simulink model "MCU_Fault"  (R2022b)
settings: Solver=FixedStepDiscrete  StartTime=0.0  StopTime=10.0  FixedStep=1e-4  RelTol=1e-3
values from neighbouring files (symbols this model uses):
  C_Fault_CntDectiontime_u32 = 0.0    [MCU_FaultDiag_Datadictionary.sldd]    (also in MCU_Fault_Datadictionary_objects.m = myPackage.Parameter; MCU_Fault_Datadictionary_objects.sldd)
  C_Fault_IaConfirmCnt_u16 = 0.0    [MCU_FaultDiag_Datadictionary.sldd]    (also in MCU_Fault_Datadictionary_objects.m = myPackage.Parameter; MCU_Fault_Datadictionary_objects.sldd)
  C_Fault_IbConfirmCnt_u16 = 0.0    [MCU_FaultDiag_Datadictionary.sldd]    (also in MCU_Fault_Datadictionary_objects.m = myPackage.Parameter; MCU_Fault_Datadictionary_objects.sldd)
  C_Fault_IbLimit_s32 = 0.0    [MCU_FaultDiag_Datadictionary.sldd]    (also in MCU_Fault_Datadictionary_objects.m = myPackage.Parameter; MCU_Fault_Datadictionary_objects.sldd)
  C_Fault_IcConfirmCnt_u16 = 0.0    [MCU_FaultDiag_Datadictionary.sldd]    (also in MCU_Fault_Datadictionary_objects.m = myPackage.Parameter; MCU_Fault_Datadictionary_objects.sldd)
  C_Fault_IcLimit_s32 = 0.0    [MCU_FaultDiag_Datadictionary.sldd]    (also in MCU_Fault_Datadictionary_objects.m = myPackage.Parameter; MCU_Fault_Datadictionary_objects.sldd)
  C_Fault_IphaseLimitStart_s32 = 0.0    [MCU_FaultDiag_Datadictionary.sldd]    (also in MCU_Fault_Datadictionary_objects.m = myPackage.Parameter; MCU_Fault_Datadictionary_objects.sldd)
  C_Fault_MotorTempSensor_i16 = 0.0    [MCU_FaultDiag_Datadictionary.sldd]    (also in MCU_Fault_Datadictionary_objects.m = myPackage.Parameter; MCU_Fault_Datadictionary_objects.sldd)
  C_Fault_SpdUpFaultConfirmCnt_u16 = 0.0    [MCU_FaultDiag_Datadictionary.sldd]    (also in MCU_Fault_Datadictionary_objects.m = myPackage.Parameter; MCU_Fault_Datadictionary_objects.sldd)
  C_Fault_SpdUpLimitStart_i16 = 0.0    [MCU_FaultDiag_Datadictionary.sldd]    (also in MCU_Fault_Datadictionary_objects.m = myPackage.Parameter; MCU_Fault_Datadictionary_objects.sldd)
  C_Fault_SpdUpLimitStop_i16 = 0.0    [MCU_FaultDiag_Datadictionary.sldd]    (also in MCU_Fault_Datadictionary_objects.m = myPackage.Parameter; MCU_Fault_Datadictionary_objects.sldd)
  C_Fault_SpdUpWarnConfirmCnt_u16 = 0.0    [MCU_FaultDiag_Datadictionary.sldd]    (also in MCU_Fault_Datadictionary_objects.m = myPackage.Parameter; MCU_Fault_Datadictionary_objects.sldd)
  C_Fault_TigbtCircutConfirmCnt_u16 = 0.0    [MCU_FaultDiag_Datadictionary.sldd]    (also in MCU_Fault_Datadictionary_objects.m = myPackage.Parameter; MCU_Fault_Datadictionary_objects.sldd)
  C_Fault_TigbtCircutConfirmTh_u16 = 0.0    [MCU_FaultDiag_Datadictionary.sldd]    (also in MCU_Fault_Datadictionary_objects.m = myPackage.Parameter; MCU_Fault_Datadictionary_objects.sldd)
  C_Fault_TigbtCircutFaultEn_u8 = 0.0    [MCU_FaultDiag_Datadictionary.sldd]    (also in MCU_Fault_Datadictionary_objects.m = myPackage.Parameter; MCU_Fault_Datadictionary_objects.sldd)
  C_Fault_TigbtLimitStart_i16 = 0.0    [MCU_FaultDiag_Datadictionary.sldd]    (also in MCU_Fault_Datadictionary_objects.m = myPackage.Parameter; MCU_Fault_Datadictionary_objects.sldd)
  C_Fault_TigbtLimitStop_i16 = 0.0    [MCU_FaultDiag_Datadictionary.sldd]    (also in MCU_Fault_Datadictionary_objects.m = myPackage.Parameter; MCU_Fault_Datadictionary_objects.sldd)
  C_Fault_TigbtOverConfirmCnt_u16 = 0.0    [MCU_FaultDiag_Datadictionary.sldd]    (also in MCU_Fault_Datadictionary_objects.m = myPackage.Parameter; MCU_Fault_Datadictionary_objects.sldd)
  C_Fault_TigbtWarnConfirmCnt_u16 = 0.0    [MCU_FaultDiag_Datadictionary.sldd]    (also in MCU_Fault_Datadictionary_objects.m = myPackage.Parameter; MCU_Fault_Datadictionary_objects.sldd)
  C_Fault_TmotorCircutConfirmCnt_u16 = 0.0    [MCU_FaultDiag_Datadictionary.sldd]    (also in MCU_Fault_Datadictionary_objects.m = myPackage.Parameter; MCU_Fault_Datadictionary_objects.sldd)
  C_Fault_TmotorCircutConfirmTh_u16 = 0.0    [MCU_FaultDiag_Datadictionary.sldd]    (also in MCU_Fault_Datadictionary_objects.m = myPackage.Parameter; MCU_Fault_Datadictionary_objects.sldd)
  C_Fault_TmotorCircutFaultEn_u8 = 0.0    [MCU_FaultDiag_Datadictionary.sldd]    (also in MCU_Fault_Datadictionary_objects.m = myPackage.Parameter; MCU_Fault_Datadictionary_objects.sldd)
  C_Fault_TmotorLimitStart_i16 = 0.0    [MCU_FaultDiag_Datadictionary.sldd]    (also in MCU_Fault_Datadictionary_objects.m = myPackage.Parameter; MCU_Fault_Datadictionary_objects.sldd)
  C_Fault_TmotorLimitStop_i16 = 0.0    [MCU_FaultDiag_Datadictionary.sldd]    (also in MCU_Fault_Datadictionary_objects.m = myPackage.Parameter; MCU_Fault_Datadictionary_objects.sldd)
  C_Fault_TmotorOverConfirmCnt_u16 = 0.0    [MCU_FaultDiag_Datadictionary.sldd]    (also in MCU_Fault_Datadictionary_objects.m = myPackage.Parameter; MCU_Fault_Datadictionary_objects.sldd)
  C_Fault_TmotorWarnConfirmCnt_u16 = 0.0    [MCU_FaultDiag_Datadictionary.sldd]    (also in MCU_Fault_Datadictionary_objects.m = myPackage.Parameter; MCU_Fault_Datadictionary_objects.sldd)
  C_Fault_UdcLoFaultConfirmCnt_u16 = 0.0    [MCU_FaultDiag_Datadictionary.sldd]    (also in MCU_Fault_Datadictionary_objects.m = myPackage.Parameter; MCU_Fault_Datadictionary_objects.sldd)
  C_Fault_UdcLoWarnConfirmCnt_u16 = 0.0    [MCU_FaultDiag_Datadictionary.sldd]    (also in MCU_Fault_Datadictionary_objects.m = myPackage.Parameter; MCU_Fault_Datadictionary_objects.sldd)
  C_Fault_UdcUpFaultConfirmCnt_u16 = 0.0    [MCU_FaultDiag_Datadictionary.sldd]    (also in MCU_Fault_Datadictionary_objects.m = myPackage.Parameter; MCU_Fault_Datadictionary_objects.sldd)
  C_Fault_UdcUpWarnConfirmCnt_u16 = 0.0    [MCU_FaultDiag_Datadictionary.sldd]    (also in MCU_Fault_Datadictionary_objects.m = myPackage.Parameter; MCU_Fault_Datadictionary_objects.sldd)
undefined symbols (not defined in the file or in its folder): AB_SAMPLE, ABC_SAMPLE, AC_SAMPLE, BC_SAMPLE, ParamCfg_LaValueDefault_u16, ParamCfg_SampleMode_u16, VEHICLE
libraries: simulink x30
(part 1 of 2)
settings Model: DataDictionary=MCU_Fault_Datadictionary_objects.sldd  Creator=ZYH  LastModifiedBy=ZYH
settings OptimizationCC: DefaultParameterBehavior=Inlined  EnhancedBackFolding=on  PassReuseOutputArgsAs=Individual arguments  ZeroExternalMemoryAtStartup=off  ZeroInternalMemoryAtStartup=off  OptimizeBlockOrder=speed  DifferentSizesBufferReuse=on  OptimizationCustomize=off  EfficientTunableParamExpr=on
settings DebuggingCC: ParameterTunabilityLossMsg=error
settings SFSimCC: MATLABDynamicMemAlloc=off
settings RTWCC: Description=Embedded Coder  SystemTargetFile=ert.tlc  GenCodeOnly=on  TemplateMakefile=ert_default_tmf
settings CodeAppCC: ForceParamTrailComments=on  IgnoreCustomStorageClasses=off  OperatorAnnotations=on  SimulinkDataObjDesc=on  SFDataObjDesc=on  InsertBlockDesc=on
settings ERTTargetCC: TargetLangStandard=C99 (ISO)  GenerateSampleERTMain=on  InlinedParameterPlacement=NonHierarchical  ERTCustomFileTemplate=example_file_process.tlc

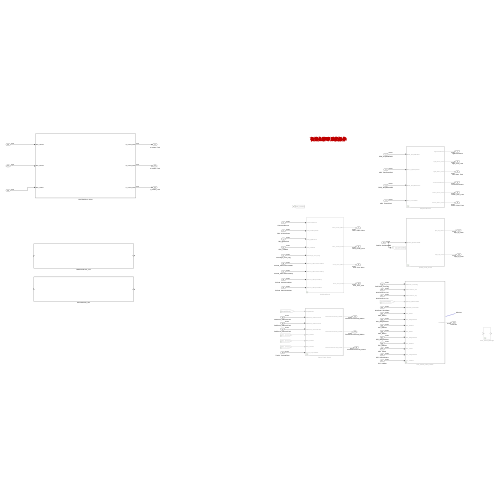
[thumbnail: Simulink's stored preview of the top-level diagram]
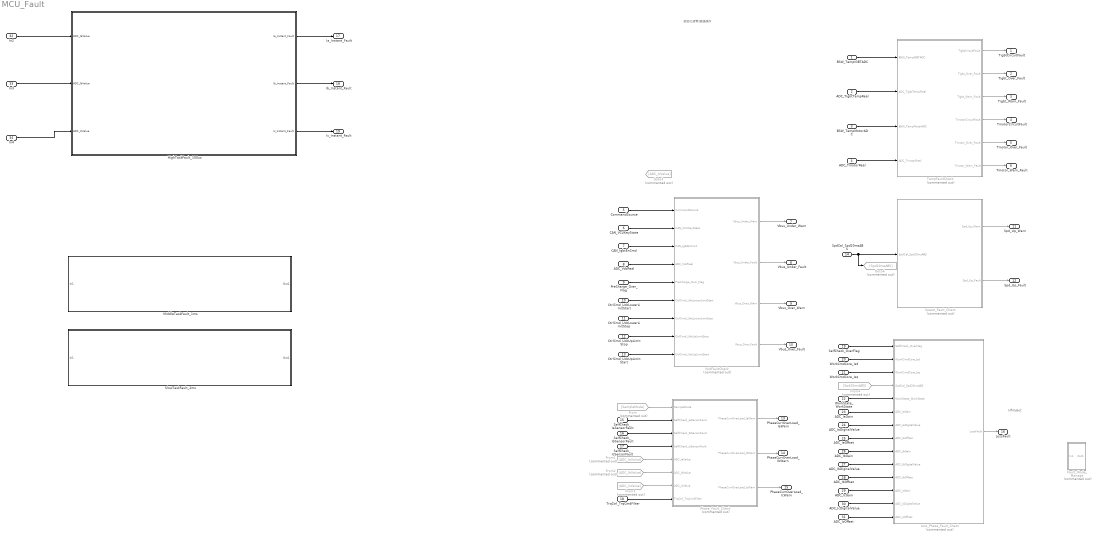
== system MCU_Fault ==
  note: 初始化清零/赋值操作
  note: HfiInJect
  BSW_TempIGBTADC : Inport
  ADC_TigbtTempReal : Inport  Port=2
  BSW_TempMotorADC : Inport  Port=3
  ADC_TmotorReal : Inport  Port=4
  CommandSource : Inport  Port=5
  CAN_VCUKeyState : Inport  Port=6
  CAN_IgbtEnCmd : Inport  Port=7
  ADC_VdcReal : Inport  Port=8
  PreCharge_Over_Flag : Inport  Port=9
  CtrlCmd_UdcLowerLimitStart : Inport  Port=10
  CtrlCmd_UdcLowerLimitStop : Inport  Port=11
  CtrlCmd_UdcUpLimitStop : Inport  Port=12
  CtrlCmd_UdcUpLimitStart : Inport  Port=13
  SpdCal_Spd20msABS : Inport  Port=14
  SelfCheck_IaSensorFault : Inport  Port=15
  SelfCheck_IbSensorFault : Inport  Port=16
  SelfCheck_IcSensorFault : Inport  Port=17
  TrqCtrl_TrqCmdFilter : Inport  Port=18
  SelfCheck_OverFlag : Inport  Port=19
  WorkCmdCore_Isd : Inport  Port=20
  WorkCmdCore_Isq : Inport  Port=21
  WorkState_WorkState : Inport  Port=22
  ADC_IaGain : Inport  Port=23
  ADC_IaDigitalValue : Inport  Port=24
  ADC_IaOffset : Inport  Port=25
  ADC_IbGain : Inport  Port=26
  ADC_IbDigitalValue : Inport  Port=27
  ADC_IbOffset : Inport  Port=28
  ADC_IcGain : Inport  Port=29
  ADC_IcDigitalValue : Inport  Port=30
  ADC_IcOffset : Inport  Port=31
  In2 : Inport  Port=32
  In3 : Inport  Port=33
  In4 : Inport  Port=34
  Fault_Mode_Manage : Subsystem  Commented=on
  From : From  Commented=on  GotoTag=SampleMode
  From1 : From  Commented=on  GotoTag=ADC_IaValue
  From2 : From  Commented=on  GotoTag=ADC_IbValue
  From3 : From  Commented=on  GotoTag=ADC_IcValue
  From4 : From  Commented=on  GotoTag=Spd20msABS
  Goto3 : Goto  Commented=on  GotoTag=ADC_IcValue
  Goto4 : Goto  Commented=on  GotoTag=Spd20msABS
  HighTaskFault_100us : Subsystem
  Lost_Phase_Fault_Check : Subsystem  Commented=on  TreatAsAtomicUnit=on
  MiddleTaskFault_1ms : Subsystem
  Phase_Fault_Check : Subsystem  Commented=on  TreatAsAtomicUnit=on
  SlowTaskFault_2ms : Subsystem
  Speed_Fault_Check : Subsystem  Commented=on  TreatAsAtomicUnit=on
  TempFaultCheck : Subsystem  Commented=on  TreatAsAtomicUnit=on
      settings: RTWSystemCode=Nonreusable function
  VoltFaultCheck : Subsystem  Commented=on
      settings: RTWSystemCode=Nonreusable function
  TigbtCircuitFault : Outport
  Tigbt_Over_Fault : Outport  Port=2
  Tigbt_Warn_Fault : Outport  Port=3
  TmotorCircuitFault : Outport  Port=4
  Tmotor_Over_Fault : Outport  Port=5
  Tmotor_Warn_Fault : Outport  Port=6
  Vbus_Under_Warn : Outport  Port=7
  Vbus_Under_Fault : Outport  Port=8
  Vbus_Over_Warn : Outport  Port=9
  Vbus_Over_Fault : Outport  Port=10
  Spd_Up_Warn : Outport  Port=11
  Spd_Up_Fault : Outport  Port=12
  PhaseCurrOverLoad_IaWarn : Outport  Port=13
  PhaseCurrOverLoad_IbWarn : Outport  Port=14
  PhaseCurrOverLoad_IcWarn : Outport  Port=15
  LossFault : Outport  Port=16
  Ia_Instant_Fault : Outport  Port=17
  Ib_Instant_Fault : Outport  Port=18
  Ic_Instant_Fault : Outport  Port=19
  wires:
  BSW_TempIGBTADC/1 -> TempFaultCheck/1(BSW_TempIGBTADC)
  ADC_TmotorReal/1 -> TempFaultCheck/4(ADC_TmotorReal)
  ADC_TigbtTempReal/1 -> TempFaultCheck/2(ADC_TigbtTempReal)
  BSW_TempMotorADC/1 -> TempFaultCheck/3(BSW_TempMotorADC)
  TempFaultCheck/1(TigbtCircuitFault) -> TigbtCircuitFault/1
  TempFaultCheck/2(Tigbt_Over_Fault) -> Tigbt_Over_Fault/1
  TempFaultCheck/3(Tigbt_Warn_Fault) -> Tigbt_Warn_Fault/1
  TempFaultCheck/4(TmotorCircuitFault) -> TmotorCircuitFault/1
  TempFaultCheck/5(Tmotor_Over_Fault) -> Tmotor_Over_Fault/1
  TempFaultCheck/6(Tmotor_Warn_Fault) -> Tmotor_Warn_Fault/1
  CommandSource/1 -> VoltFaultCheck/1(CommandSource)
  CAN_VCUKeyState/1 -> VoltFaultCheck/2(CAN_VCUKeyState)
  CAN_IgbtEnCmd/1 -> VoltFaultCheck/3(CAN_IgbtEnCmd)
  ADC_VdcReal/1 -> VoltFaultCheck/4(ADC_VdcReal)
  PreCharge_Over_Flag/1 -> VoltFaultCheck/5(PreCharge_Over_Flag)
  CtrlCmd_UdcLowerLimitStart/1 -> VoltFaultCheck/6(CtrlCmd_UdcLowerLimitStart)
  CtrlCmd_UdcLowerLimitStop/1 -> VoltFaultCheck/7(CtrlCmd_UdcLowerLimitStop)
  CtrlCmd_UdcUpLimitStop/1 -> VoltFaultCheck/8(CtrlCmd_UdcUpLimitStop)
  CtrlCmd_UdcUpLimitStart/1 -> VoltFaultCheck/9(CtrlCmd_UdcUpLimitStart)
  VoltFaultCheck/1(Vbus_Under_Warn) -> Vbus_Under_Warn/1
  VoltFaultCheck/2(Vbus_Under_Fault) -> Vbus_Under_Fault/1
  VoltFaultCheck/3(Vbus_Over_Warn) -> Vbus_Over_Warn/1
  VoltFaultCheck/4(Vbus_Over_Fault) -> Vbus_Over_Fault/1
  SpdCal_Spd20msABS/1 -> Speed_Fault_Check/1(SpdCal_Spd20msABS), Goto4/1
  Speed_Fault_Check/1(Spd_Up_Warn) -> Spd_Up_Warn/1
  Speed_Fault_Check/2(Spd_Up_Fault) -> Spd_Up_Fault/1
  SelfCheck_IaSensorFault/1 -> Phase_Fault_Check/2(SelfCheck_IaSensorFault)
  SelfCheck_IbSensorFault/1 -> Phase_Fault_Check/3(SelfCheck_IbSensorFault)
  SelfCheck_IcSensorFault/1 -> Phase_Fault_Check/4(SelfCheck_IcSensorFault)
  From/1 -> Phase_Fault_Check/1(SampleMode)
  From1/1 -> Phase_Fault_Check/5(ADC_IaValue)
  From2/1 -> Phase_Fault_Check/6(ADC_IbValue)
  From3/1 -> Phase_Fault_Check/7(ADC_IcValue)
  TrqCtrl_TrqCmdFilter/1 -> Phase_Fault_Check/8(TrqCtrl_TrqCmdFilter)
  Phase_Fault_Check/1(PhaseCurrOverLoad_IaWarn) -> PhaseCurrOverLoad_IaWarn/1
  Phase_Fault_Check/2(PhaseCurrOverLoad_IbWarn) -> PhaseCurrOverLoad_IbWarn/1
  Phase_Fault_Check/3(PhaseCurrOverLoad_IcWarn) -> PhaseCurrOverLoad_IcWarn/1
  SelfCheck_OverFlag/1 -> Lost_Phase_Fault_Check/1(SelfCheck_OverFlag)
  WorkCmdCore_Isd/1 -> Lost_Phase_Fault_Check/2(WorkCmdCore_Isd)
  WorkCmdCore_Isq/1 -> Lost_Phase_Fault_Check/3(WorkCmdCore_Isq)
  From4/1 -> Lost_Phase_Fault_Check/4(SpdCal_Spd20msABS)
  WorkState_WorkState/1 -> Lost_Phase_Fault_Check/5(WorkState_WorkState)
  ADC_IaGain/1 -> Lost_Phase_Fault_Check/6(ADC_IaGain)
  ADC_IaDigitalValue/1 -> Lost_Phase_Fault_Check/7(ADC_IaDigitalValue)
  ADC_IaOffset/1 -> Lost_Phase_Fault_Check/8(ADC_IaOffset)
  ADC_IbGain/1 -> Lost_Phase_Fault_Check/9(ADC_IbGain)
  ADC_IbDigitalValue/1 -> Lost_Phase_Fault_Check/10(ADC_IbDigitalValue)
  ADC_IbOffset/1 -> Lost_Phase_Fault_Check/11(ADC_IbOffset)
  ADC_IcGain/1 -> Lost_Phase_Fault_Check/12(ADC_IcGain)
  ADC_IcDigitalValue/1 -> Lost_Phase_Fault_Check/13(ADC_IcDigitalValue)
  ADC_IcOffset/1 -> Lost_Phase_Fault_Check/14(ADC_IcOffset)
  Lost_Phase_Fault_Check/1(LossFault) -> LossFault/1
  In3/1 -> HighTaskFault_100us/2(ADC_IbValue)
  In4/1 -> HighTaskFault_100us/3(ADC_IcValue)
  In2/1 -> HighTaskFault_100us/1(ADC_IaValue)
  HighTaskFault_100us/3(Ic_Instant_Fault) -> Ic_Instant_Fault/1
  HighTaskFault_100us/2(Ib_Instant_Fault) -> Ib_Instant_Fault/1
  HighTaskFault_100us/1(Ia_Instant_Fault) -> Ia_Instant_Fault/1

== system MCU_Fault/Fault_Mode_Manage ==
  In1 : Inport
  Out1 : Outport
  wires:
  In1/1 -> Out1/1

== system MCU_Fault/HighTaskFault_100us ==
  ADC_IaValue : Inport
  ADC_IbValue : Inport  Port=2
  ADC_IcValue : Inport  Port=3
  Constant : Constant  Value=ParamCfg_SampleMode_u16
  InterruptFaultCheck_100us : Subsystem  TreatAsAtomicUnit=on
      settings: RTWSystemCode=Nonreusable function
  Ia_Instant_Fault : Outport
  Ib_Instant_Fault : Outport  Port=2
  Ic_Instant_Fault : Outport  Port=3
  wires:
  ADC_IcValue/1 -> InterruptFaultCheck_100us/4(ADC_IcValue)
  ADC_IbValue/1 -> InterruptFaultCheck_100us/3(ADC_IbValue)
  ADC_IaValue/1 -> InterruptFaultCheck_100us/2(ADC_IaValue)
  InterruptFaultCheck_100us/1(Ia_Instant_Fault) -> Ia_Instant_Fault/1
  InterruptFaultCheck_100us/2(Ib_Instant_Fault) -> Ib_Instant_Fault/1
  InterruptFaultCheck_100us/3(Ic_Instant_Fault) -> Ic_Instant_Fault/1
  Constant/1 -> InterruptFaultCheck_100us/1(SampleMode)

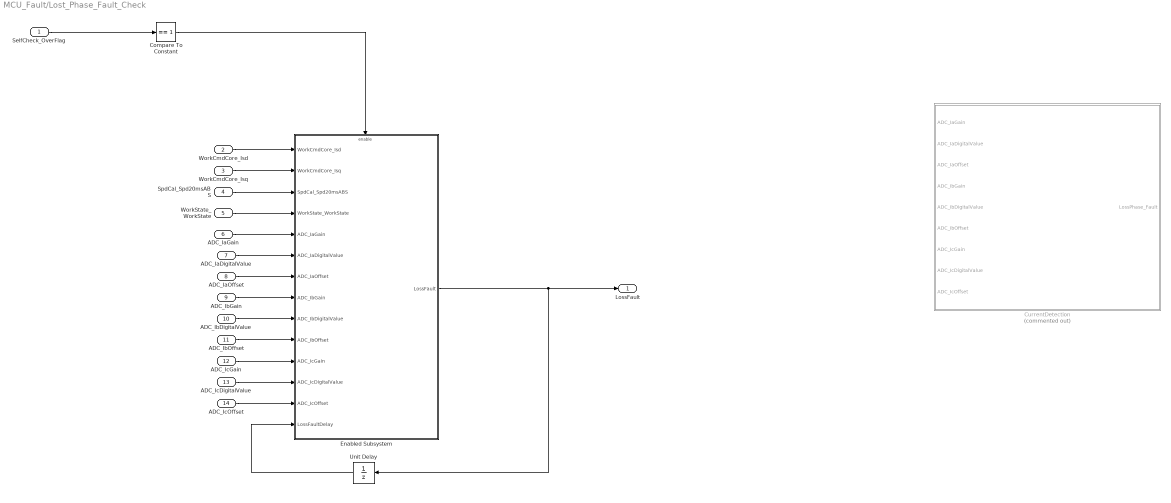
== system MCU_Fault/Lost_Phase_Fault_Check ==
  SelfCheck_OverFlag : Inport
  WorkCmdCore_Isd : Inport  Port=2
  WorkCmdCore_Isq : Inport  Port=3
  SpdCal_Spd20msABS : Inport  Port=4
  WorkState_WorkState : Inport  Port=5
  ADC_IaGain : Inport  Port=6
  ADC_IaDigitalValue : Inport  Port=7
  ADC_IaOffset : Inport  Port=8
  ADC_IbGain : Inport  Port=9
  ADC_IbDigitalValue : Inport  Port=10
  ADC_IbOffset : Inport  Port=11
  ADC_IcGain : Inport  Port=12
  ADC_IcDigitalValue : Inport  Port=13
  ADC_IcOffset : Inport  Port=14
  Compare To Constant : simulink/Logic and Bit Operations/Compare To Constant  relop===  const=1  OutDataTypeStr=boolean
  CurrentDetection : Subsystem  Commented=on
  Enabled Subsystem : Subsystem  TreatAsAtomicUnit=on
  Unit Delay : UnitDelay  SampleTime=-1  HasFrameUpgradeWarning=on
  LossFault : Outport
  wires:
  SelfCheck_OverFlag/1 -> Compare To Constant/1
  Compare To Constant/1 -> Enabled Subsystem/Enable
  Enabled Subsystem/1(LossFault) -> LossFault/1, Unit Delay/1
  Unit Delay/1 -> Enabled Subsystem/14(LossFaultDelay)
  WorkCmdCore_Isd/1 -> Enabled Subsystem/1(WorkCmdCore_Isd)
  WorkCmdCore_Isq/1 -> Enabled Subsystem/2(WorkCmdCore_Isq)
  SpdCal_Spd20msABS/1 -> Enabled Subsystem/3(SpdCal_Spd20msABS)
  WorkState_WorkState/1 -> Enabled Subsystem/4(WorkState_WorkState)
  ADC_IaGain/1 -> Enabled Subsystem/5(ADC_IaGain)
  ADC_IaDigitalValue/1 -> Enabled Subsystem/6(ADC_IaDigitalValue)
  ADC_IaOffset/1 -> Enabled Subsystem/7(ADC_IaOffset)
  ADC_IbGain/1 -> Enabled Subsystem/8(ADC_IbGain)
  ADC_IbDigitalValue/1 -> Enabled Subsystem/9(ADC_IbDigitalValue)
  ADC_IbOffset/1 -> Enabled Subsystem/10(ADC_IbOffset)
  ADC_IcGain/1 -> Enabled Subsystem/11(ADC_IcGain)
  ADC_IcDigitalValue/1 -> Enabled Subsystem/12(ADC_IcDigitalValue)
  ADC_IcOffset/1 -> Enabled Subsystem/13(ADC_IcOffset)

== system MCU_Fault/MiddleTaskFault_1ms ==
  In1 : Inport
  Out1 : Outport
  wires:
  In1/1 -> Out1/1

== system MCU_Fault/Phase_Fault_Check ==
  SampleMode : Inport
  SelfCheck_IaSensorFault : Inport  Port=2
  SelfCheck_IbSensorFault : Inport  Port=3
  SelfCheck_IcSensorFault : Inport  Port=4
  ADC_IaValue : Inport  Port=5
  ADC_IbValue : Inport  Port=6
  ADC_IcValue : Inport  Port=7
  TrqCtrl_TrqCmdFilter : Inport  Port=8
  Compare To Zero : simulink/Logic and Bit Operations/Compare To Zero  relop===  OutDataTypeStr=boolean
  Compare To Zero1 : simulink/Logic and Bit Operations/Compare To Zero  relop===  OutDataTypeStr=boolean
  Compare To Zero2 : simulink/Logic and Bit Operations/Compare To Zero  relop===  OutDataTypeStr=boolean
  Logical Operator3 : Logic  Inputs=3  AllPortsSameDT=off  OutDataTypeStr=boolean
  Subsystem : Subsystem
  PhaseCurrOverLoad_IaWarn : Outport
  PhaseCurrOverLoad_IbWarn : Outport  Port=2
  PhaseCurrOverLoad_IcWarn : Outport  Port=3
  wires:
  SelfCheck_IaSensorFault/1 -> Compare To Zero/1  "M_Fault_IaSensorFault_u8"
  SelfCheck_IbSensorFault/1 -> Compare To Zero1/1  "M_Fault_IbSensorFault_u8"
  SelfCheck_IcSensorFault/1 -> Compare To Zero2/1  "M_Fault_IcSensorFault_u8"
  Compare To Zero/1 -> Logical Operator3/1
  Compare To Zero1/1 -> Logical Operator3/2
  Compare To Zero2/1 -> Logical Operator3/3
  SampleMode/1 -> Subsystem/1(SampleMode)
  Logical Operator3/1 -> Subsystem/Enable
  ADC_IaValue/1 -> Subsystem/2(ADC_IaValue)
  ADC_IbValue/1 -> Subsystem/3(ADC_IbValue)
  ADC_IcValue/1 -> Subsystem/4(ADC_IcValue)
  TrqCtrl_TrqCmdFilter/1 -> Subsystem/5(TrqCtrl_TrqCmdFilter)  "M_Fault_TrqCmdFilter_s32"
  Subsystem/1(PhaseCurrOverLoad_IaWarn) -> PhaseCurrOverLoad_IaWarn/1
  Subsystem/2(PhaseCurrOverLoad_IbWarn) -> PhaseCurrOverLoad_IbWarn/1
  Subsystem/3(PhaseCurrOverLoad_IcWarn) -> PhaseCurrOverLoad_IcWarn/1

== system MCU_Fault/SlowTaskFault_2ms ==
  In1 : Inport
  Out1 : Outport
  wires:
  In1/1 -> Out1/1

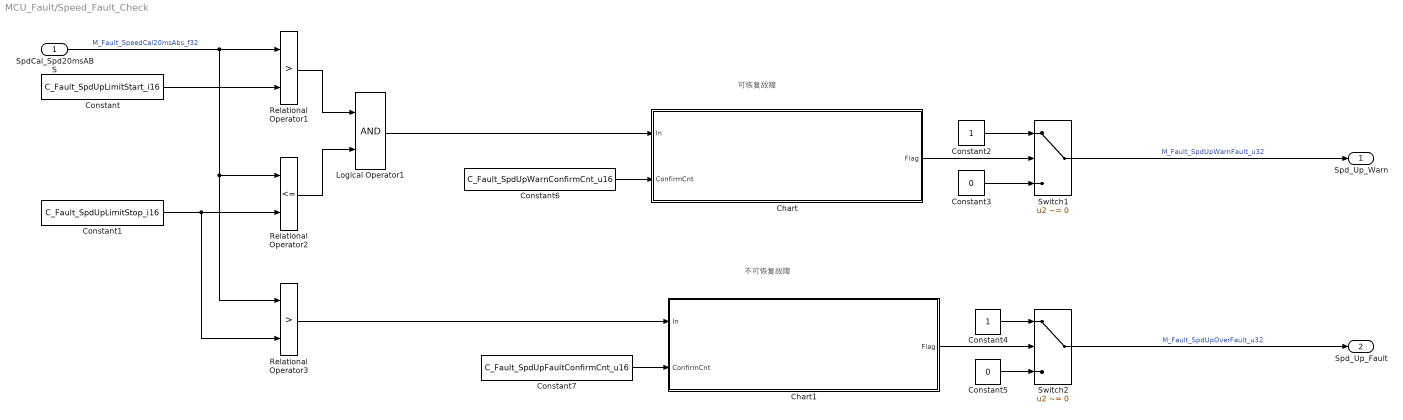
== system MCU_Fault/Speed_Fault_Check ==
  note: 不可恢复故障
  note: 可恢复故障
  SpdCal_Spd20msABS : Inport
  Chart : Stateflow chart  TreatAsAtomicUnit=on
  Chart1 : Stateflow chart  TreatAsAtomicUnit=on
  Constant : Constant  Value=C_Fault_SpdUpLimitStart_i16
  Constant1 : Constant  Value=C_Fault_SpdUpLimitStop_i16
  Constant2 : Constant  OutDataTypeStr=uint32
  Constant3 : Constant  Value=0  OutDataTypeStr=uint32
  Constant4 : Constant  OutDataTypeStr=uint32
  Constant5 : Constant  Value=0  OutDataTypeStr=uint32
  Constant6 : Constant  Value=C_Fault_SpdUpWarnConfirmCnt_u16
  Constant7 : Constant  Value=C_Fault_SpdUpFaultConfirmCnt_u16
  Logical Operator1 : Logic  AllPortsSameDT=off  OutDataTypeStr=boolean
  Relational Operator1 : RelationalOperator  Operator=>  OutDataTypeStr=boolean  RndMeth=Simplest  InputSameDT=off
  Relational Operator2 : RelationalOperator  Operator=<=  OutDataTypeStr=boolean  RndMeth=Simplest  InputSameDT=off
  Relational Operator3 : RelationalOperator  Operator=>  OutDataTypeStr=boolean  RndMeth=Simplest  InputSameDT=off
  Switch1 : Switch  Criteria=u2 ~= 0  SaturateOnIntegerOverflow=off  InputSameDT=off
  Switch2 : Switch  Criteria=u2 ~= 0  SaturateOnIntegerOverflow=off  InputSameDT=off
  Spd_Up_Warn : Outport
  Spd_Up_Fault : Outport  Port=2
  wires:
  Logical Operator1/1 -> Chart/1(In)
  Switch2/1 -> Spd_Up_Fault/1  "M_Fault_SpdUpOverFault_u32"
  Relational Operator3/1 -> Chart1/1(In)
  Constant5/1 -> Switch2/3
  Switch1/1 -> Spd_Up_Warn/1  "M_Fault_SpdUpWarnFault_u32"
  Chart1/1(Flag) -> Switch2/2
  Constant4/1 -> Switch2/1
  Relational Operator1/1 -> Logical Operator1/1
  Constant7/1 -> Chart1/2(ConfirmCnt)
  Constant1/1 -> Relational Operator3/2, Relational Operator2/2
  Constant6/1 -> Chart/2(ConfirmCnt)
  Constant3/1 -> Switch1/3
  SpdCal_Spd20msABS/1 -> Relational Operator3/1, Relational Operator2/1, Relational Operator1/1  "M_Fault_SpeedCal20msAbs_f32"
  Chart/1(Flag) -> Switch1/2
  Constant2/1 -> Switch1/1
  Constant/1 -> Relational Operator1/2
  Relational Operator2/1 -> Logical Operator1/2

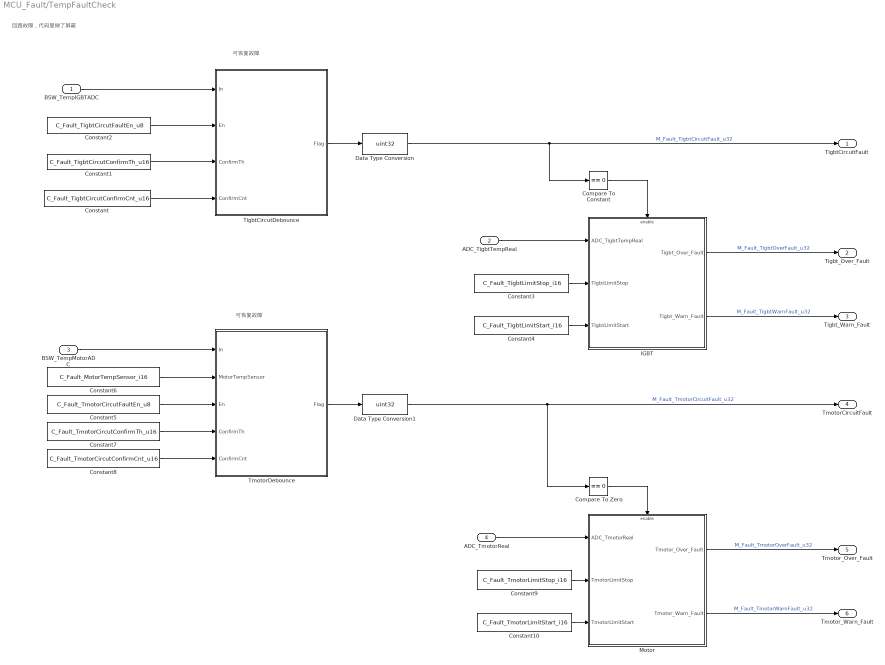
== system MCU_Fault/TempFaultCheck ==
  note: 回路故障，代码里做了屏蔽
  note: 可恢复故障
  note: 可恢复故障
  BSW_TempIGBTADC : Inport
  ADC_TigbtTempReal : Inport  Port=2
  BSW_TempMotorADC : Inport  Port=3
  ADC_TmotorReal : Inport  Port=4
  Compare To Constant : simulink/Logic and Bit Operations/Compare To Constant  relop===  const=0  OutDataTypeStr=boolean
  Compare To Zero : simulink/Logic and Bit Operations/Compare To Zero  relop===  OutDataTypeStr=boolean
  Constant : Constant  Value=C_Fault_TigbtCircutConfirmCnt_u16  OutDataTypeStr=uint16
  Constant1 : Constant  Value=C_Fault_TigbtCircutConfirmTh_u16  OutDataTypeStr=uint16
  Constant10 : Constant  Value=C_Fault_TmotorLimitStart_i16  OutDataTypeStr=int16
  Constant2 : Constant  Value=C_Fault_TigbtCircutFaultEn_u8  OutDataTypeStr=uint8
  Constant3 : Constant  Value=C_Fault_TigbtLimitStop_i16  OutDataTypeStr=int16
  Constant4 : Constant  Value=C_Fault_TigbtLimitStart_i16  OutDataTypeStr=int16
  Constant5 : Constant  Value=C_Fault_TmotorCircutFaultEn_u8  OutDataTypeStr=uint8
  Constant6 : Constant  Value=C_Fault_MotorTempSensor_i16  OutDataTypeStr=int16
  Constant7 : Constant  Value=C_Fault_TmotorCircutConfirmTh_u16  OutDataTypeStr=uint16
  Constant8 : Constant  Value=C_Fault_TmotorCircutConfirmCnt_u16  OutDataTypeStr=uint16
  Constant9 : Constant  Value=C_Fault_TmotorLimitStop_i16  OutDataTypeStr=int16
  Data Type Conversion : DataTypeConversion  OutDataTypeStr=uint32  SaturateOnIntegerOverflow=off  RndMeth=Floor
  Data Type Conversion1 : DataTypeConversion  OutDataTypeStr=uint32  SaturateOnIntegerOverflow=off  RndMeth=Floor
  IGBT : Subsystem  TreatAsAtomicUnit=on
  Motor : Subsystem  TreatAsAtomicUnit=on
  TigbtCircutDebounce : Stateflow chart  TreatAsAtomicUnit=on
      settings: PortSchema="{\"entries\":[{\"content\":{\"sides\":[{\"content\":{\"connectorIds\":[\"In2\",\"In4\",\"In3\",\"In1\"]},\"type\":\"ConnectorPlacement.EquallySpacedRectSide\",\"uuid\":\"cb643c20-0648-4de0-95a0-2dc0cea02081\"},{\"content\":{\"connectorIds\":[\"Out1\"],\"side\":\"RIGHT\"},\"type\":\"ConnectorPlacement.EquallySpacedRectSide\",\"uuid\":\"2b2785c0-bbb5-46d9-9c97-4314d513a69a\"},{\"content\":{\"connectorIds\":[],\"side\":\"TOP\"},\"type\":\"ConnectorPlacement.EquallySpacedRectSide\",\"uuid\":\"79ac1ab1-637b-4565-8653-1b1baa55e4cd\"}]},\"type\":\"ConnectorPlacement.EquallySpacedConnector\",\"uuid\":\"b76854ae-8754-44d0-b8b9-3a13cdedbdf9\"}],\"packageUris\":[\"http://schema.mathworks.com/mf0/Connector/R2020b\"],\"version\":\"1.0\"}"
  TmotorDebounce : Stateflow chart  TreatAsAtomicUnit=on
      settings: PortSchema="{\"entries\":[{\"content\":{\"sides\":[{\"content\":{\"connectorIds\":[\"In3\",\"In2\",\"In5\",\"In4\",\"In1\"]},\"type\":\"ConnectorPlacement.EquallySpacedRectSide\",\"uuid\":\"cb643c20-0648-4de0-95a0-2dc0cea02081\"},{\"content\":{\"connectorIds\":[\"Out1\"],\"side\":\"RIGHT\"},\"type\":\"ConnectorPlacement.EquallySpacedRectSide\",\"uuid\":\"2b2785c0-bbb5-46d9-9c97-4314d513a69a\"},{\"content\":{\"connectorIds\":[],\"side\":\"TOP\"},\"type\":\"ConnectorPlacement.EquallySpacedRectSide\",\"uuid\":\"79ac1ab1-637b-4565-8653-1b1baa55e4cd\"}]},\"type\":\"ConnectorPlacement.EquallySpacedConnector\",\"uuid\":\"b76854ae-8754-44d0-b8b9-3a13cdedbdf9\"}],\"packageUris\":[\"http://schema.mathworks.com/mf0/Connector/R2020b\"],\"version\":\"1.0\"}"
  TigbtCircuitFault : Outport
  Tigbt_Over_Fault : Outport  Port=2
  Tigbt_Warn_Fault : Outport  Port=3
  TmotorCircuitFault : Outport  Port=4
  Tmotor_Over_Fault : Outport  Port=5
  Tmotor_Warn_Fault : Outport  Port=6
  wires:
  Constant1/1 -> TigbtCircutDebounce/3(ConfirmTh)
  Constant/1 -> TigbtCircutDebounce/1(ConfirmCnt)
  Constant2/1 -> TigbtCircutDebounce/4(En)
  BSW_TempIGBTADC/1 -> TigbtCircutDebounce/2(In)
  TigbtCircutDebounce/1(Flag) -> Data Type Conversion/1
  Data Type Conversion/1 -> Compare To Constant/1, TigbtCircuitFault/1  "M_Fault_TigbtCircuitFault_u32"
  Compare To Constant/1 -> IGBT/Enable
  Constant3/1 -> IGBT/2(TigbtLimitStop)
  Constant4/1 -> IGBT/3(TigbtLimitStart)
  ADC_TigbtTempReal/1 -> IGBT/1(ADC_TigbtTempReal)
  IGBT/1(Tigbt_Over_Fault) -> Tigbt_Over_Fault/1  "M_Fault_TigbtOverFault_u32"
  IGBT/2(Tigbt_Warn_Fault) -> Tigbt_Warn_Fault/1  "M_Fault_TigbtWarnFault_u32"
  BSW_TempMotorADC/1 -> TmotorDebounce/3(In)
  Constant6/1 -> TmotorDebounce/2(MotorTempSensor)
  Constant5/1 -> TmotorDebounce/5(En)
  Constant8/1 -> TmotorDebounce/1(ConfirmCnt)
  Constant7/1 -> TmotorDebounce/4(ConfirmTh)
  TmotorDebounce/1(Flag) -> Data Type Conversion1/1
  Data Type Conversion1/1 -> Compare To Zero/1, TmotorCircuitFault/1  "M_Fault_TmotorCircuitFault_u32"
  Compare To Zero/1 -> Motor/Enable
  ADC_TmotorReal/1 -> Motor/1(ADC_TmotorReal)
  Constant9/1 -> Motor/2(TmotorLimitStop)
  Constant10/1 -> Motor/3(TmotorLimitStart)
  Motor/1(Tmotor_Over_Fault) -> Tmotor_Over_Fault/1  "M_Fault_TmotorOverFault_u32"
  Motor/2(Tmotor_Warn_Fault) -> Tmotor_Warn_Fault/1  "M_Fault_TmotorWarnFault_u32"

== system MCU_Fault/VoltFaultCheck ==
  note: 不做成标定量是因为
      | 代码里区分了Analog模式和其他模式下的欠过压阈值
  CommandSource : Inport
  CAN_VCUKeyState : Inport  Port=2
  CAN_IgbtEnCmd : Inport  Port=3
  ADC_VdcReal : Inport  Port=4
  PreCharge_Over_Flag : Inport  Port=5
  CtrlCmd_UdcLowerLimitStart : Inport  Port=6
  CtrlCmd_UdcLowerLimitStop : Inport  Port=7
  CtrlCmd_UdcUpLimitStop : Inport  Port=8
  CtrlCmd_UdcUpLimitStart : Inport  Port=9
  VdcLowerFaultCheck : Subsystem  TreatAsAtomicUnit=on
  VdcOverFaultCheck : Subsystem  TreatAsAtomicUnit=on
  Vbus_Under_Warn : Outport
  Vbus_Under_Fault : Outport  Port=2
  Vbus_Over_Warn : Outport  Port=3
  Vbus_Over_Fault : Outport  Port=4
  wires:
  CommandSource/1 -> VdcLowerFaultCheck/1(CommandSource)  "M_Fault_CommandSource_i16"
  CAN_VCUKeyState/1 -> VdcLowerFaultCheck/2(CAN_VCUKeyState)  "M_Fault_VCUKeyState_u16"
  CAN_IgbtEnCmd/1 -> VdcLowerFaultCheck/3(CAN_IgbtEnCmd)  "M_Fault_IgbtEnCmd_u16"
  PreCharge_Over_Flag/1 -> VdcLowerFaultCheck/4(PreCharge_Over_Flag)  "M_Fault_PrechargeOverFlg_u16"
  ADC_VdcReal/1 -> VdcOverFaultCheck/1(ADC_VdcReal), VdcLowerFaultCheck/5(ADC_VdcReal)  "M_Fault_UdcReal_s32"
  CtrlCmd_UdcLowerLimitStart/1 -> VdcLowerFaultCheck/6(CtrlCmd_UdcLowerLimitStart)  "M_Fault_UdcLowerLimitStart_s32"
  CtrlCmd_UdcLowerLimitStop/1 -> VdcLowerFaultCheck/7(CtrlCmd_UdcLowerLimitStop)  "M_Fault_UdcLowerLimitStop_s32"
  VdcLowerFaultCheck/1(Vbus_Under_Warn) -> Vbus_Under_Warn/1  "M_Fault_VdcUnderWarn_u32"
  VdcLowerFaultCheck/2(Vbus_Under_Fault) -> Vbus_Under_Fault/1  "M_Fault_VdcUnderFault_u32"
  CtrlCmd_UdcUpLimitStop/1 -> VdcOverFaultCheck/3(CtrlCmd_UdcUpLimitStop)  "M_Fault_UdcUpLimitStop_s32"
  CtrlCmd_UdcUpLimitStart/1 -> VdcOverFaultCheck/2(CtrlCmd_UdcUpLimitStart)  "M_Fault_UdcUpLimitStart_s32"
  VdcOverFaultCheck/1(Vbus_Over_Warn) -> Vbus_Over_Warn/1  "M_Fault_UdcUpWarn_u32"
  VdcOverFaultCheck/2(Vbus_Over_Fault) -> Vbus_Over_Fault/1  "M_Fault_UdcUpFault_u32"

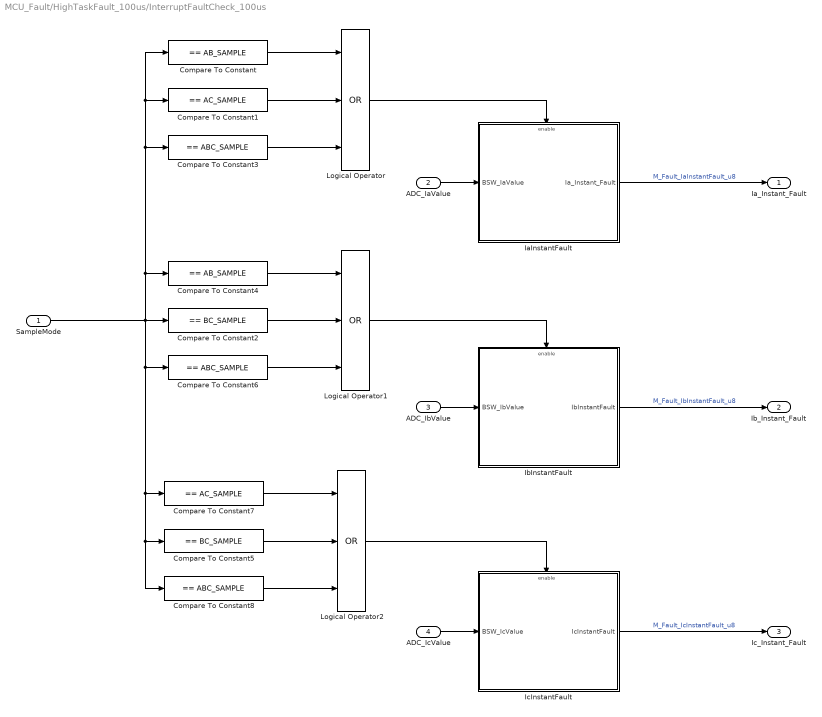
== system MCU_Fault/HighTaskFault_100us/InterruptFaultCheck_100us ==
  SampleMode : Inport
  ADC_IaValue : Inport  Port=2
  ADC_IbValue : Inport  Port=3
  ADC_IcValue : Inport  Port=4
  Compare To Constant : simulink/Logic and Bit Operations/Compare To Constant  relop===  const=AB_SAMPLE  OutDataTypeStr=boolean
  Compare To Constant1 : simulink/Logic and Bit Operations/Compare To Constant  relop===  const=AC_SAMPLE  OutDataTypeStr=boolean
  Compare To Constant2 : simulink/Logic and Bit Operations/Compare To Constant  relop===  const=BC_SAMPLE  OutDataTypeStr=boolean
  Compare To Constant3 : simulink/Logic and Bit Operations/Compare To Constant  relop===  const=ABC_SAMPLE  OutDataTypeStr=boolean
  Compare To Constant4 : simulink/Logic and Bit Operations/Compare To Constant  relop===  const=AB_SAMPLE  OutDataTypeStr=boolean
  Compare To Constant5 : simulink/Logic and Bit Operations/Compare To Constant  relop===  const=BC_SAMPLE  OutDataTypeStr=boolean
  Compare To Constant6 : simulink/Logic and Bit Operations/Compare To Constant  relop===  const=ABC_SAMPLE  OutDataTypeStr=boolean
  Compare To Constant7 : simulink/Logic and Bit Operations/Compare To Constant  relop===  const=AC_SAMPLE  OutDataTypeStr=boolean
  Compare To Constant8 : simulink/Logic and Bit Operations/Compare To Constant  relop===  const=ABC_SAMPLE  OutDataTypeStr=boolean
  IaInstantFault : Subsystem  TreatAsAtomicUnit=on
  IbInstantFault : Subsystem  TreatAsAtomicUnit=on
  IcInstantFault : Subsystem  TreatAsAtomicUnit=on
  Logical Operator : Logic  Operator=OR  Inputs=3  AllPortsSameDT=off  OutDataTypeStr=boolean
  Logical Operator1 : Logic  Operator=OR  Inputs=3  AllPortsSameDT=off  OutDataTypeStr=boolean
  Logical Operator2 : Logic  Operator=OR  Inputs=3  AllPortsSameDT=off  OutDataTypeStr=boolean
  Ia_Instant_Fault : Outport
  Ib_Instant_Fault : Outport  Port=2
  Ic_Instant_Fault : Outport  Port=3
  wires:
  SampleMode/1 -> Compare To Constant/1, Compare To Constant1/1, Compare To Constant3/1, Compare To Constant4/1, Compare To Constant8/1, Compare To Constant5/1, Compare To Constant7/1, Compare To Constant6/1, Compare To Constant2/1
  Compare To Constant/1 -> Logical Operator/1
  Compare To Constant1/1 -> Logical Operator/2
  Compare To Constant3/1 -> Logical Operator/3
  Logical Operator/1 -> IaInstantFault/Enable
  ADC_IaValue/1 -> IaInstantFault/1(BSW_IaValue)
  Compare To Constant6/1 -> Logical Operator1/3
  Compare To Constant2/1 -> Logical Operator1/2
  Compare To Constant4/1 -> Logical Operator1/1
  Logical Operator1/1 -> IbInstantFault/Enable
  ADC_IbValue/1 -> IbInstantFault/1(BSW_IbValue)
  Compare To Constant5/1 -> Logical Operator2/2
  Compare To Constant7/1 -> Logical Operator2/1
  Compare To Constant8/1 -> Logical Operator2/3
  Logical Operator2/1 -> IcInstantFault/Enable
  ADC_IcValue/1 -> IcInstantFault/1(BSW_IcValue)
  IaInstantFault/1(Ia_Instant_Fault) -> Ia_Instant_Fault/1  "M_Fault_IaInstantFault_u8"
  IbInstantFault/1(IbInstantFault) -> Ib_Instant_Fault/1  "M_Fault_IbInstantFault_u8"
  IcInstantFault/1(IcInstantFault) -> Ic_Instant_Fault/1  "M_Fault_IcInstantFault_u8"

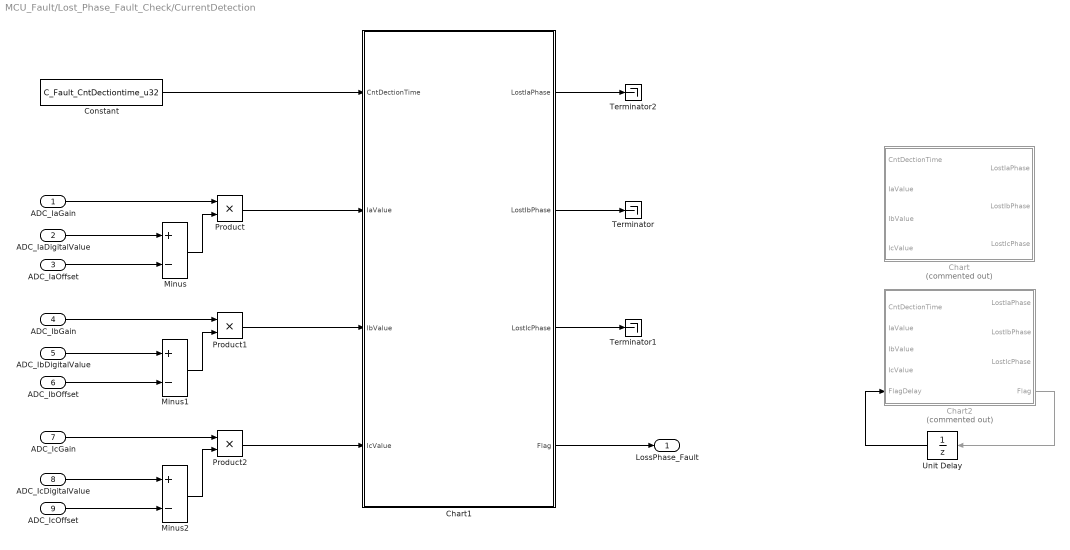
== system MCU_Fault/Lost_Phase_Fault_Check/CurrentDetection ==
  ADC_IaGain : Inport
  ADC_IaDigitalValue : Inport  Port=2
  ADC_IaOffset : Inport  Port=3
  ADC_IbGain : Inport  Port=4
  ADC_IbDigitalValue : Inport  Port=5
  ADC_IbOffset : Inport  Port=6
  ADC_IcGain : Inport  Port=7
  ADC_IcDigitalValue : Inport  Port=8
  ADC_IcOffset : Inport  Port=9
  Chart : Stateflow chart  Commented=on  TreatAsAtomicUnit=on
  Chart1 : Stateflow chart  TreatAsAtomicUnit=on
  Chart2 : Stateflow chart  Commented=on  TreatAsAtomicUnit=on
      settings: PortSchema="{\"entries\":[{\"content\":{\"sides\":[{\"content\":{\"connectorIds\":[\"In2\",\"In3\",\"In4\",\"In5\",\"In1\"]},\"type\":\"ConnectorPlacement.EquallySpacedRectSide\",\"uuid\":\"7ee51362-cc53-4c4b-bb72-7e7d7fdfa368\"},{\"content\":{\"connectorIds\":[\"Out1\",\"Out2\",\"Out3\",\"Out4\"],\"side\":\"RIGHT\"},\"type\":\"ConnectorPlacement.EquallySpacedRectSide\",\"uuid\":\"f10f55d3-9130-490d-9732-47c24a5d1591\"},{\"content\":{\"connectorIds\":[],\"side\":\"TOP\"},\"type\":\"ConnectorPlacement.EquallySpacedRectSide\",\"uuid\":\"d4ead924-d192-479a-942e-9c33d44277d2\"},{\"content\":{\"connectorIds\":[],\"side\":\"BOTTOM\"},\"type\":\"ConnectorPlacement.EquallySpacedRectSide\",\"uuid\":\"0567de3f-c1c5-4c0c-81d8-e5bcc3ace347\"}]},\"type\":\"ConnectorPlacement.EquallySpacedConnector\",\"uuid\":\"51e6a2cf-dee8-429b-a62c-1b7f30850334\"}],\"packageUris\":[\"http://schema.mathworks.com/mf0/Connector/R2020b\"],\"version\":\"1.0\"}"
  Constant : Constant  Value=C_Fault_CntDectiontime_u32
  Minus : Sum  Inputs=+-
  Minus1 : Sum  Inputs=+-
  Minus2 : Sum  Inputs=+-
  Product : Product
  Product1 : Product
  Product2 : Product
  Terminator : Terminator
  Terminator1 : Terminator
  Terminator2 : Terminator
  Unit Delay : UnitDelay  SampleTime=-1  HasFrameUpgradeWarning=on
  LossPhase_Fault : Outport
  wires:
  ADC_IaDigitalValue/1 -> Minus/1
  ADC_IaOffset/1 -> Minus/2
  ADC_IaGain/1 -> Product/1
  Minus/1 -> Product/2
  Product/1 -> Chart1/2(IaValue)
  ADC_IbDigitalValue/1 -> Minus1/1
  ADC_IbOffset/1 -> Minus1/2
  ADC_IbGain/1 -> Product1/1
  Minus1/1 -> Product1/2
  ADC_IcDigitalValue/1 -> Minus2/1
  ADC_IcOffset/1 -> Minus2/2
  ADC_IcGain/1 -> Product2/1
  Minus2/1 -> Product2/2
  Product1/1 -> Chart1/3(IbValue)
  Product2/1 -> Chart1/4(IcValue)
  Constant/1 -> Chart1/1(CntDectionTime)
  Chart1/2(LostIbPhase) -> Terminator/1
  Chart1/3(LostIcPhase) -> Terminator1/1
  Chart1/1(LostIaPhase) -> Terminator2/1
  Chart1/4(Flag) -> LossPhase_Fault/1
  Chart2/4(Flag) -> Unit Delay/1
  Unit Delay/1 -> Chart2/1(FlagDelay)

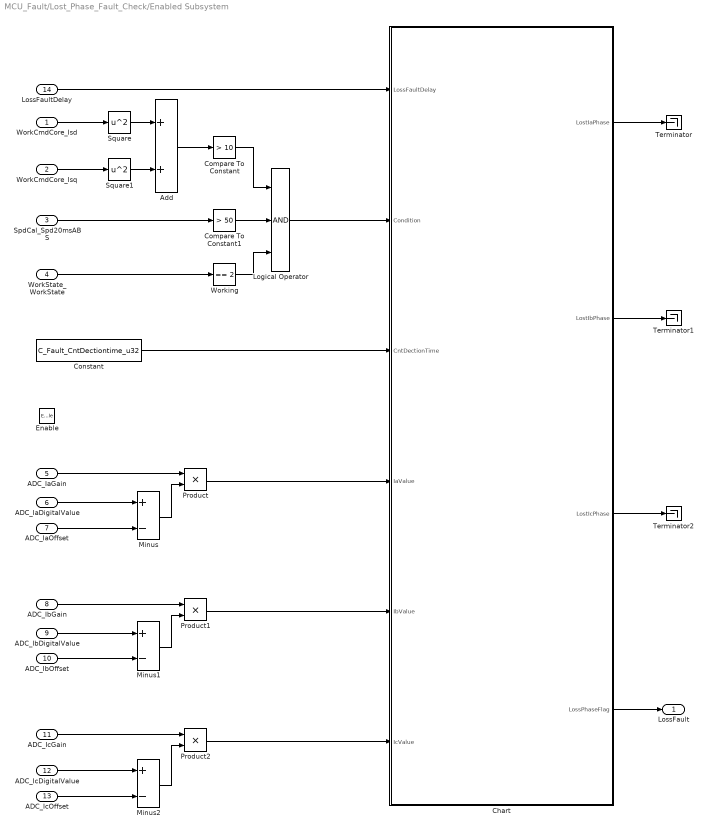
== system MCU_Fault/Lost_Phase_Fault_Check/Enabled Subsystem ==
  WorkCmdCore_Isd : Inport
  WorkCmdCore_Isq : Inport  Port=2
  SpdCal_Spd20msABS : Inport  Port=3
  WorkState_WorkState : Inport  Port=4
  ADC_IaGain : Inport  Port=5
  ADC_IaDigitalValue : Inport  Port=6
  ADC_IaOffset : Inport  Port=7
  ADC_IbGain : Inport  Port=8
  ADC_IbDigitalValue : Inport  Port=9
  ADC_IbOffset : Inport  Port=10
  ADC_IcGain : Inport  Port=11
  ADC_IcDigitalValue : Inport  Port=12
  ADC_IcOffset : Inport  Port=13
  LossFaultDelay : Inport  Port=14
  Enable : EnablePort
  Add : Sum
  Chart : Stateflow chart  TreatAsAtomicUnit=on
  Compare To Constant : simulink/Logic and Bit Operations/Compare To Constant  relop=>  const=10  OutDataTypeStr=boolean
  Compare To Constant1 : simulink/Logic and Bit Operations/Compare To Constant  relop=>  const=50  OutDataTypeStr=boolean
  Constant : Constant  Value=C_Fault_CntDectiontime_u32
  Logical Operator : Logic  Inputs=3  AllPortsSameDT=off  OutDataTypeStr=boolean
  Minus : Sum  Inputs=+-
  Minus1 : Sum  Inputs=+-
  Minus2 : Sum  Inputs=+-
  Product : Product
  Product1 : Product
  Product2 : Product
  Square : Math  Operator=square
  Square1 : Math  Operator=square
  Terminator : Terminator
  Terminator1 : Terminator
  Terminator2 : Terminator
  Working : simulink/Logic and Bit Operations/Compare To Constant  relop===  const=2  OutDataTypeStr=boolean
  LossFault : Outport
  wires:
  LossFaultDelay/1 -> Chart/1(LossFaultDelay)
  WorkCmdCore_Isd/1 -> Square/1
  WorkCmdCore_Isq/1 -> Square1/1
  Square/1 -> Add/1
  Square1/1 -> Add/2
  Add/1 -> Compare To Constant/1
  SpdCal_Spd20msABS/1 -> Compare To Constant1/1
  WorkState_WorkState/1 -> Working/1
  Compare To Constant1/1 -> Logical Operator/2
  Compare To Constant/1 -> Logical Operator/1
  Working/1 -> Logical Operator/3
  Logical Operator/1 -> Chart/2(Condition)
  Product/1 -> Chart/4(IaValue)
  Product2/1 -> Chart/6(IcValue)
  ADC_IaDigitalValue/1 -> Minus/1
  ADC_IcGain/1 -> Product2/1
  Product1/1 -> Chart/5(IbValue)
  ADC_IaOffset/1 -> Minus/2
  Minus1/1 -> Product1/2
  ADC_IaGain/1 -> Product/1
  ADC_IbOffset/1 -> Minus1/2
  ADC_IcOffset/1 -> Minus2/2
  Minus/1 -> Product/2
  ADC_IbDigitalValue/1 -> Minus1/1
  Minus2/1 -> Product2/2
  ADC_IcDigitalValue/1 -> Minus2/1
  ADC_IbGain/1 -> Product1/1
  Constant/1 -> Chart/3(CntDectionTime)
  Chart/1(LostIaPhase) -> Terminator/1
  Chart/2(LostIbPhase) -> Terminator1/1
  Chart/3(LostIcPhase) -> Terminator2/1
  Chart/4(LossPhaseFlag) -> LossFault/1

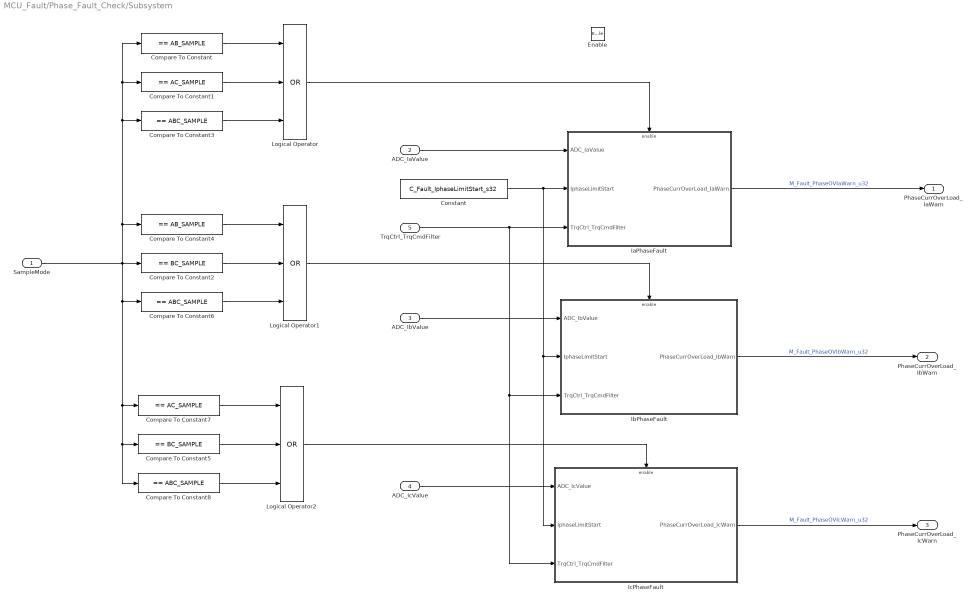
== system MCU_Fault/Phase_Fault_Check/Subsystem ==
  SampleMode : Inport
  ADC_IaValue : Inport  Port=2
  ADC_IbValue : Inport  Port=3
  ADC_IcValue : Inport  Port=4
  TrqCtrl_TrqCmdFilter : Inport  Port=5
  Enable : EnablePort
  Compare To Constant : simulink/Logic and Bit Operations/Compare To Constant  relop===  const=AB_SAMPLE  OutDataTypeStr=boolean
  Compare To Constant1 : simulink/Logic and Bit Operations/Compare To Constant  relop===  const=AC_SAMPLE  OutDataTypeStr=boolean
  Compare To Constant2 : simulink/Logic and Bit Operations/Compare To Constant  relop===  const=BC_SAMPLE  OutDataTypeStr=boolean
  Compare To Constant3 : simulink/Logic and Bit Operations/Compare To Constant  relop===  const=ABC_SAMPLE  OutDataTypeStr=boolean
  Compare To Constant4 : simulink/Logic and Bit Operations/Compare To Constant  relop===  const=AB_SAMPLE  OutDataTypeStr=boolean
  Compare To Constant5 : simulink/Logic and Bit Operations/Compare To Constant  relop===  const=BC_SAMPLE  OutDataTypeStr=boolean
  Compare To Constant6 : simulink/Logic and Bit Operations/Compare To Constant  relop===  const=ABC_SAMPLE  OutDataTypeStr=boolean
  Compare To Constant7 : simulink/Logic and Bit Operations/Compare To Constant  relop===  const=AC_SAMPLE  OutDataTypeStr=boolean
  Compare To Constant8 : simulink/Logic and Bit Operations/Compare To Constant  relop===  const=ABC_SAMPLE  OutDataTypeStr=boolean
  Constant : Constant  Value=C_Fault_IphaseLimitStart_s32
  IaPhaseFault : Subsystem  TreatAsAtomicUnit=on
  IbPhaseFault : Subsystem  TreatAsAtomicUnit=on
  IcPhaseFault : Subsystem  TreatAsAtomicUnit=on
  Logical Operator : Logic  Operator=OR  Inputs=3  AllPortsSameDT=off  OutDataTypeStr=boolean
  Logical Operator1 : Logic  Operator=OR  Inputs=3  AllPortsSameDT=off  OutDataTypeStr=boolean
  Logical Operator2 : Logic  Operator=OR  Inputs=3  AllPortsSameDT=off  OutDataTypeStr=boolean
  PhaseCurrOverLoad_IaWarn : Outport
  PhaseCurrOverLoad_IbWarn : Outport  Port=2
  PhaseCurrOverLoad_IcWarn : Outport  Port=3
  wires:
  Compare To Constant7/1 -> Logical Operator2/1
  Compare To Constant8/1 -> Logical Operator2/3
  Compare To Constant1/1 -> Logical Operator/2
  Compare To Constant/1 -> Logical Operator/1
  SampleMode/1 -> Compare To Constant/1, Compare To Constant1/1, Compare To Constant3/1, Compare To Constant4/1, Compare To Constant8/1, Compare To Constant5/1, Compare To Constant7/1, Compare To Constant6/1, Compare To Constant2/1
  Compare To Constant4/1 -> Logical Operator1/1
  Compare To Constant6/1 -> Logical Operator1/3
  Compare To Constant2/1 -> Logical Operator1/2
  Compare To Constant3/1 -> Logical Operator/3
  Compare To Constant5/1 -> Logical Operator2/2
  Logical Operator/1 -> IaPhaseFault/Enable
  Logical Operator2/1 -> IcPhaseFault/Enable
  Logical Operator1/1 -> IbPhaseFault/Enable
  ADC_IaValue/1 -> IaPhaseFault/1(ADC_IaValue)
  Constant/1 -> IcPhaseFault/2(IphaseLimitStart), IbPhaseFault/2(IphaseLimitStart), IaPhaseFault/2(IphaseLimitStart)
  TrqCtrl_TrqCmdFilter/1 -> IcPhaseFault/3(TrqCtrl_TrqCmdFilter), IbPhaseFault/3(TrqCtrl_TrqCmdFilter), IaPhaseFault/3(TrqCtrl_TrqCmdFilter)
  ADC_IbValue/1 -> IbPhaseFault/1(ADC_IbValue)
  ADC_IcValue/1 -> IcPhaseFault/1(ADC_IcValue)
  IaPhaseFault/1(PhaseCurrOverLoad_IaWarn) -> PhaseCurrOverLoad_IaWarn/1  "M_Fault_PhaseOVIaWarn_u32"
  IbPhaseFault/1(PhaseCurrOverLoad_IbWarn) -> PhaseCurrOverLoad_IbWarn/1  "M_Fault_PhaseOVIbWarn_u32"
  IcPhaseFault/1(PhaseCurrOverLoad_IcWarn) -> PhaseCurrOverLoad_IcWarn/1  "M_Fault_PhaseOVIcWarn_u32"

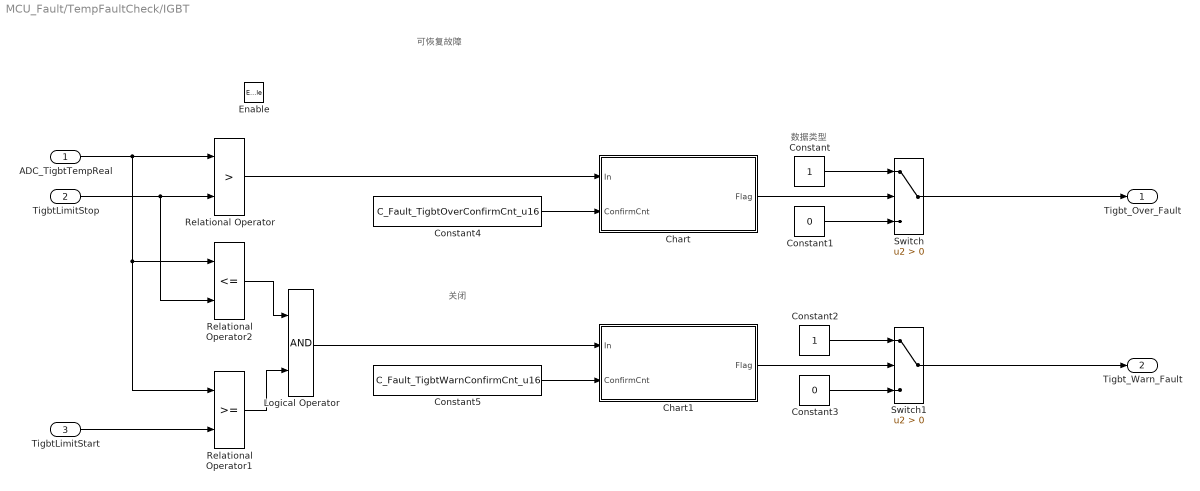
== system MCU_Fault/TempFaultCheck/IGBT ==
  note: 关闭
  note: 数据类型
  note: 可恢复故障
  ADC_TigbtTempReal : Inport
  TigbtLimitStop : Inport  Port=2
  TigbtLimitStart : Inport  Port=3
  Enable : EnablePort
  Chart : Stateflow chart  TreatAsAtomicUnit=on
  Chart1 : Stateflow chart  TreatAsAtomicUnit=on
  Constant : Constant  OutDataTypeStr=uint32
  Constant1 : Constant  Value=0  OutDataTypeStr=uint32
  Constant2 : Constant  OutDataTypeStr=uint32
  Constant3 : Constant  Value=0  OutDataTypeStr=uint32
  Constant4 : Constant  Value=C_Fault_TigbtOverConfirmCnt_u16
  Constant5 : Constant  Value=C_Fault_TigbtWarnConfirmCnt_u16
  Logical Operator : Logic  AllPortsSameDT=off  OutDataTypeStr=boolean
  Relational Operator : RelationalOperator  Operator=>  OutDataTypeStr=boolean  RndMeth=Simplest  InputSameDT=off
  Relational Operator1 : RelationalOperator  OutDataTypeStr=boolean  RndMeth=Simplest  InputSameDT=off
  Relational Operator2 : RelationalOperator  Operator=<=  OutDataTypeStr=boolean  RndMeth=Simplest  InputSameDT=off
  Switch : Switch  Criteria=u2 > Threshold  SaturateOnIntegerOverflow=off  InputSameDT=off
  Switch1 : Switch  Criteria=u2 > Threshold  SaturateOnIntegerOverflow=off  InputSameDT=off
  Tigbt_Over_Fault : Outport
  Tigbt_Warn_Fault : Outport  Port=2
  wires:
  ADC_TigbtTempReal/1 -> Relational Operator2/1, Relational Operator1/1, Relational Operator/1
  TigbtLimitStop/1 -> Relational Operator2/2, Relational Operator/2
  Constant/1 -> Switch/1
  Constant1/1 -> Switch/3
  Switch/1 -> Tigbt_Over_Fault/1
  TigbtLimitStart/1 -> Relational Operator1/2
  Constant2/1 -> Switch1/1
  Constant3/1 -> Switch1/3
  Switch1/1 -> Tigbt_Warn_Fault/1
  Relational Operator2/1 -> Logical Operator/1
  Relational Operator1/1 -> Logical Operator/2
  Relational Operator/1 -> Chart/1(In)
  Constant4/1 -> Chart/2(ConfirmCnt)
  Chart/1(Flag) -> Switch/2
  Constant5/1 -> Chart1/2(ConfirmCnt)
  Logical Operator/1 -> Chart1/1(In)
  Chart1/1(Flag) -> Switch1/2
